simulink model "DCCONTROL"  (R2026a)
settings: Solver=VariableStepAuto  StopTime=30
model workspace (MAT data in the model file):
  B = 0.1
  J = 0.01
  Kb = 0.01
  Kt = 0.01
  La = 0.5
  R = 1
settings Model: Creator=Kratos  LastModifiedBy=Kratos

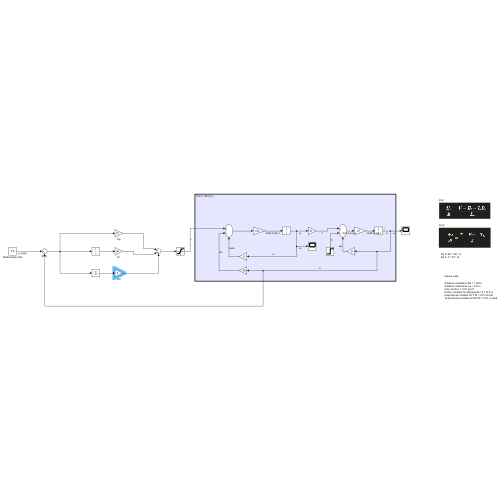
[thumbnail: Simulink's stored preview of the top-level diagram]
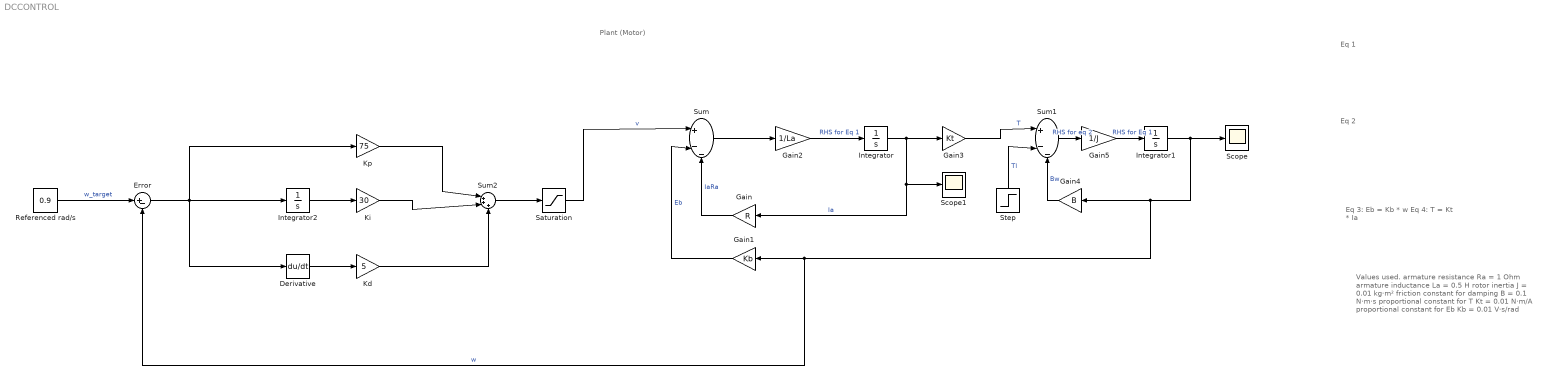
== system DCCONTROL ==
  note: Plant (Motor)
  note: Eq 3: Eb = Kb * w
      | Eq 4: T = Kt * Ia
  note: Eq 2
  note: Eq 1
  note: Values used.
      |
      | armature resistance Ra = 1 Ohm
      | armature inductance La = 0.5 H
      | rotor inertia J = 0.01 kg·m²
      | friction constant for damping B = 0.1 N·m·s
      | proportional constant for T Kt = 0.01 N·m/A
      | proportional constant for Eb Kb = 0.01 V·s/rad
  Derivative : Derivative
  Error : Sum  Inputs=|+-
  Gain : Gain  Gain=R
  Gain1 : Gain  Gain=Kb
  Gain2 : Gain  Gain=1/La
  Gain3 : Gain  Gain=Kt
  Gain4 : Gain  Gain=B
  Gain5 : Gain  Gain=1/J
  Integrator : Integrator
  Integrator1 : Integrator
  Integrator2 : Integrator
  Kd : Gain  Gain=5
  Ki : Gain  Gain=30
  Kp : Gain  Gain=75
  Referenced rad/s : Constant  Value=0.9
  Saturation : Saturate  UpperLimit=15  LowerLimit=0
  Scope : Scope
      settings: ActiveDisplayYMinimum=0.645419827478292  ActiveDisplayYMaximum=1.1466264733938636
  Scope1 : Scope
      settings: ActiveDisplayYMinimum=7.62200048882176  ActiveDisplayYMaximum=17.321722542300883
  Step : Step  Time=2  FinalValue=0.05  SampleTime=0
  Sum : Sum  Inputs=|+--
  Sum1 : Sum  Inputs=|+--
  Sum2 : Sum  Inputs=|+++
  wires:
  Integrator/1 -> Gain/1, Scope1/1, Gain3/1  "Ia"
  Gain/1 -> Sum/3  "IaRa"
  Gain1/1 -> Sum/2  "Eb"
  Sum/1 -> Gain2/1
  Gain2/1 -> Integrator/1  "RHS for Eq 1"
  Gain3/1 -> Sum1/1  "T"
  Sum1/1 -> Gain5/1  "RHS for eq 2"
  Integrator1/1 -> Scope/1, Gain1/1, Error/2, Gain4/1  "w"
  Gain4/1 -> Sum1/3  "Bw"
  Step/1 -> Sum1/2  "Tl"
  Gain5/1 -> Integrator1/1  "RHS for Eq 1"
  Referenced rad/s/1 -> Error/1  "w_target"
  Error/1 -> Derivative/1, Kp/1, Integrator2/1
  Integrator2/1 -> Ki/1
  Derivative/1 -> Kd/1
  Kd/1 -> Sum2/3
  Kp/1 -> Sum2/1
  Ki/1 -> Sum2/2
  Sum2/1 -> Saturation/1
  Saturation/1 -> Sum/1  "v"
